simulink model "tempController"  (R2019a)
settings: Solver=ode3  StartTime=0.0  StopTime=800  RelTol=1e-3
libraries: arduino_io_lib x4
settings Model: ExtModeTrigDuration=2  Creator=gcampa  LastModifiedBy=User
settings DataIOCC: LimitDataPoints=on  SaveFormat=Array  ReturnWorkspaceOutputs=off
settings OptimizationCC: LifeSpan=1
settings DebuggingCC: UnderspecifiedInitializationDetection=Classic  MergeDetectMultiDrivingBlocksExec=none  SFUnexpectedBacktrackingDiag=warning  SFNoUnconditionalDefaultTransitionDiag=warning  SFExecutionAtInitializationDiag=none  ArithmeticOperatorsInVariantConditions=warning
settings HardwareCC: ProdBitPerInt=16  ProdBitPerPointer=16  ProdBitPerSizeT=16  ProdBitPerPtrDiffT=16  ProdLargestAtomicFloat=None  ProdWordSize=8  ProdHWDeviceType=Atmel->AVR
settings ModelReferenceCC: PropagateSignalLabelsOutOfModel=off
settings SFSimCC: SimUseLocalCustomCode=off  MATLABDynamicMemAlloc=off
settings RTWCC: SystemTargetFile=realtime.tlc  GenerateMakefile=off  TemplateMakefile=realtime.tmf  Description=Run on Target Hardware  RTWVerbose=off  RTWUseLocalCustomCode=off
settings CodeAppCC: StateflowObjectComments=on
settings STFCustomTargetCC: TargetLibSuffix=.a  GenerateSampleERTMain=on  ERTCustomFileBanners=on  SupportNonInlinedSFcns=off  RemoveResetFunc=on  SupportVariableSizeSignals=on  MATLABClassNameForMDSCustomization=Simulink.SoftwareTarget.ERTCustomization  GRTInterface=off  SystemTargetFile=realtime.tlc
settings ERTTargetCC: MultiwordLength=2048  GenerateSampleERTMain=on  ParMdlRefBuildCompliant=off  CompOptLevelCompliant=off  ConcurrentExecutionCompliant=off  CombineOutputUpdateFcns=off  SupportContinuousTime=on  SupportVariableSizeSignals=on  ModelStepFunctionPrototypeControlCompliant=off  CPPClassGenCompliant=off  UseToolchainInfoCompliant=off  ExtModeTransport=3  ExtModeMexFile=ext_serial_win32_comm  ExtModeMexArgs=0 1 9600  ERTSrcFileBannerTemplate=realtime_code_template.cgt  ERTHdrFileBannerTemplate=realtime_code_template.cgt  ERTDataSrcFileTemplate=realtime_code_template.cgt  ERTDataHdrFileTemplate=realtime_code_template.cgt  ERTCustomFileTemplate=realtime_file_process.tlc  ConvertIfToSwitch=off  SuppressUnreachableDefaultCases=off
settings ConfigComp: CovMetricSettings=dw  CovHtmlReporting=on  CovSaveCumulativeToWorkspaceVar=on  CovSaveSingleToWorkspaceVar=on  CovExternalEMLEnable=off

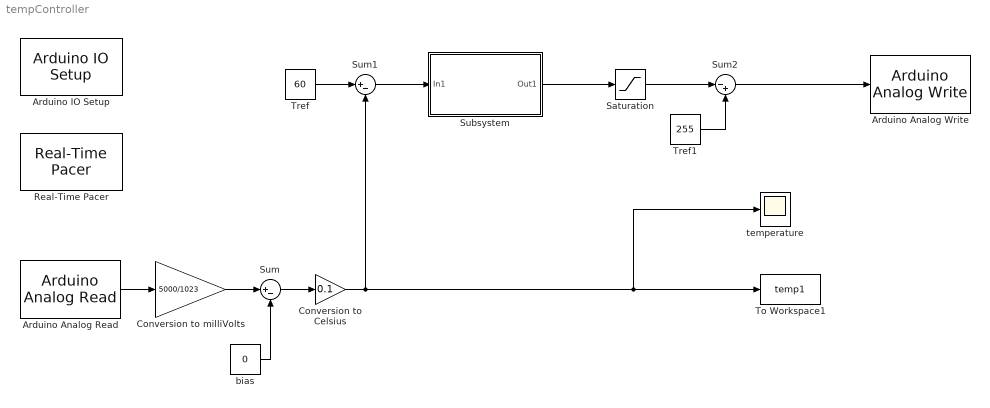
== system tempController ==
  Arduino Analog Read : arduino_io_lib/Arduino Analog Read  arduinoVar=Temporary arduino variable: Arduino1  arduinoPin=0  T=1
  Arduino Analog Write : arduino_io_lib/Arduino Analog Write  arduinoVar=Temporary arduino variable: Arduino1  arduinoPin=9  T=1
  Arduino IO Setup : arduino_io_lib/Arduino IO Setup  Priority=3  arduinoVar=Temporary arduino variable: Arduino1  workspaceVarName=b  comPort=COM5
  Conversion to Celsius : Gain  Gain=0.1
  Conversion to milliVolts : Gain  Gain=5000/1023
  Real-Time Pacer : arduino_io_lib/Real-Time Pacer  simTimePerRealTime=1
  Saturation : Saturate  UpperLimit=255  LowerLimit=0
  Subsystem : Subsystem
  Sum : Sum  Inputs=|+-
  Sum1 : Sum  Inputs=|+-
  Sum2 : Sum  Inputs=|-+
  To Workspace1 : ToWorkspace  VariableName=temp1  SaveFormat=Timeseries  SampleTime=-1
  Tref : Constant  Value=60
  Tref1 : Constant  Value=255
  bias : Constant  Value=0
  temperature : Scope
  wires:
  Conversion to milliVolts/1 -> Sum/1
  Sum/1 -> Conversion to Celsius/1
  bias/1 -> Sum/2
  Tref/1 -> Sum1/1
  Saturation/1 -> Sum2/1
  Sum2/1 -> Arduino Analog Write/1
  Conversion to Celsius/1 -> To Workspace1/1, temperature/1, Sum1/2
  Tref1/1 -> Sum2/2
  Arduino Analog Read/1 -> Conversion to milliVolts/1
  Sum1/1 -> Subsystem/1(In1)
  Subsystem/1(Out1) -> Saturation/1

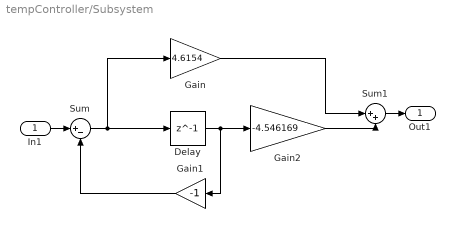
== system tempController/Subsystem ==
  In1 : Inport
  Delay : Delay  DelayLength=1  SampleTime=1
  Gain : Gain  Gain=4.6154
  Gain1 : Gain  Gain=-1
  Gain2 : Gain  Gain=-4.546169
  Sum : Sum  Inputs=|+-
  Sum1 : Sum  Inputs=|++
  Out1 : Outport
  wires:
  In1/1 -> Sum/1
  Gain2/1 -> Sum1/2
  Sum1/1 -> Out1/1
  Sum/1 -> Gain/1, Delay/1
  Gain1/1 -> Sum/2
  Gain/1 -> Sum1/1
  Delay/1 -> Gain1/1, Gain2/1
